simulink model "Nonlinear_compensator_regulate_position"  (R2021b)
settings: Solver=VariableStepAuto  StartTime=0.0  StopTime=10.0  RelTol=1e-3
values from neighbouring files (symbols this model uses):
  g = 9.81    [init.m]
  K = acker(A, B, P)    [Synthesis.m]
  Kr = 1/evalfr(posTf, 0)    [Synthesis.m]
  L = 2    [init.m]
  L_obs = temp'    [Synthesis.m]
  M = 5    [init.m]
  m = 1    [init.m]
  theta = pi    (= 3.14159265359)    [Synthesis.m]
  theta_perturbed = theta0 - perturbation    (= 2.99159265359)    [Linearization_comparison.m]    (also in Synthesis.m)
undefined symbols (not defined in the file or in its folder): A, B, C
settings Model: Creator=brizio  LastModifiedBy=brizio

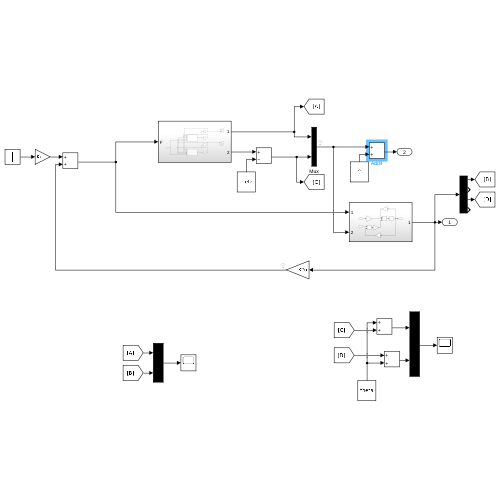
[thumbnail: Simulink's stored preview of the top-level diagram]
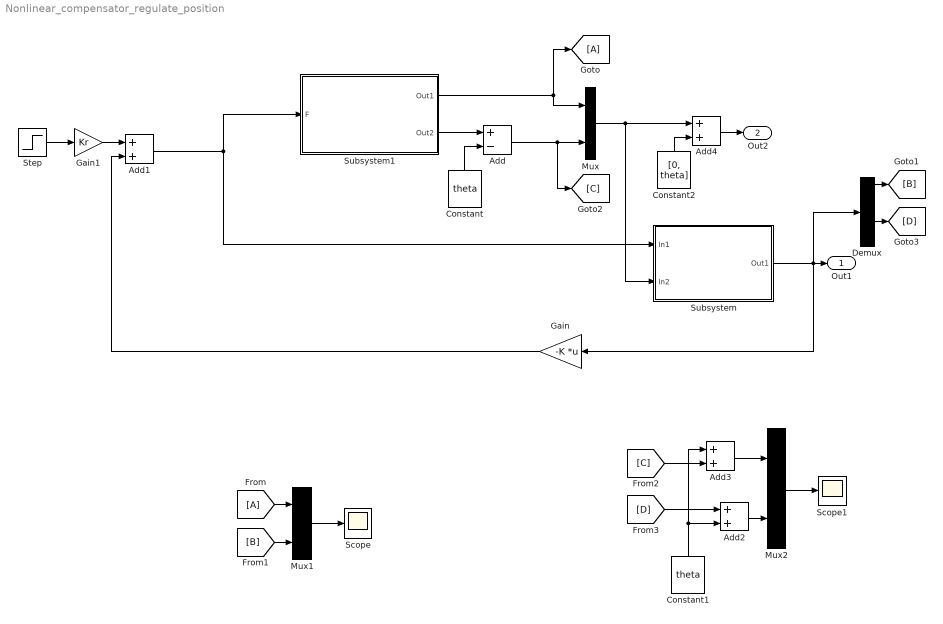
== system Nonlinear_compensator_regulate_position ==
  Add : Sum  Inputs=+-
  Add{1..4} (4 alike) : Sum
  Constant : Constant  Value=theta
  Constant1 : Constant  Value=theta
  Constant2 : Constant  Value=[0, theta]
  Demux : Demux
  Gain : Gain  Gain=-K  Multiplication=Matrix(K*u)
  Gain1 : Gain  Gain=Kr
  Mux : Mux  Inputs=2
  Mux1 : Mux  Inputs=2
  Mux2 : Mux  Inputs=2
  Scope : Scope
  Scope1 : Scope
  Step : Step  SampleTime=0
  Subsystem : Subsystem
  Subsystem1 : Subsystem
  Out1 : Outport
  Out2 : Outport  Port=2
  wires:
  Constant/1 -> Add/2
  Add2/1 -> Mux2/2
  [C] -> Add3/2
  [A] -> Mux1/1
  Add1/1 -> Subsystem1/1(F), Subsystem/1(In1)
  Add3/1 -> Mux2/1
  [B] -> Mux1/2
  Subsystem1/1(Out1) -> [A], Mux/1
  Add/1 -> [C], Mux/2
  Mux/1 -> Add4/1, Subsystem/2(In2)
  Demux/1 -> [B]
  Mux2/1 -> Scope1/1
  Subsystem/1(Out1) -> Gain/1, Out1/1, Demux/1
  [D] -> Add2/1
  Constant1/1 -> Add2/2, Add3/1
  Gain/1 -> Add1/2
  Subsystem1/2(Out2) -> Add/1
  Demux/3 -> [D]
  Mux1/1 -> Scope/1
  Gain1/1 -> Add1/1
  Step/1 -> Gain1/1
  Constant2/1 -> Add4/2
  Add4/1 -> Out2/1

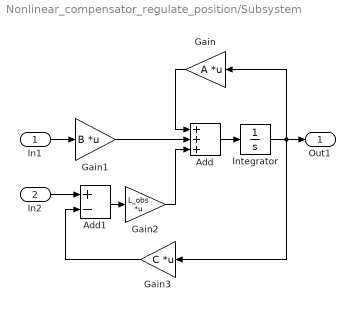
== system Nonlinear_compensator_regulate_position/Subsystem ==
  In1 : Inport
  In2 : Inport  Port=2
  Add : Sum  Inputs=+++
  Add1 : Sum  Inputs=+-
  Gain : Gain  Gain=A  Multiplication=Matrix(K*u)
  Gain1 : Gain  Gain=B  Multiplication=Matrix(K*u)
  Gain2 : Gain  Gain=L_obs  Multiplication=Matrix(K*u)
  Gain3 : Gain  Gain=C  Multiplication=Matrix(K*u)
  Integrator : Integrator
  Out1 : Outport
  wires:
  Add/1 -> Integrator/1
  In1/1 -> Gain1/1
  Gain/1 -> Add/1
  Gain1/1 -> Add/2
  Gain2/1 -> Add/3
  Add1/1 -> Gain2/1
  In2/1 -> Add1/1
  Gain3/1 -> Add1/2
  Integrator/1 -> Gain3/1, Gain/1, Out1/1

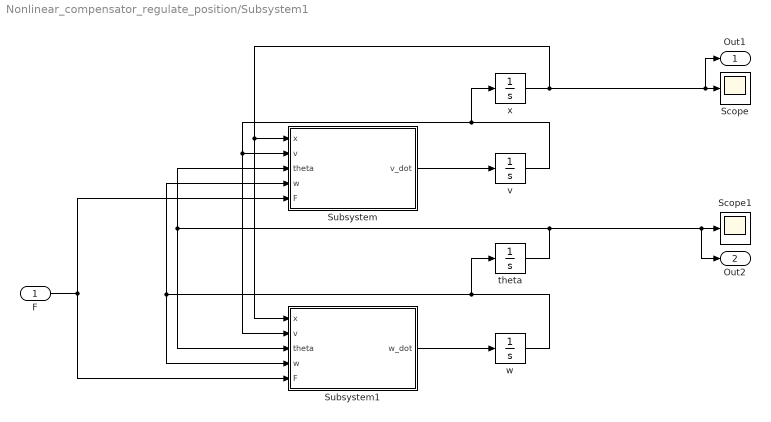
== system Nonlinear_compensator_regulate_position/Subsystem1 ==
  F : Inport
  Scope : Scope
  Scope1 : Scope
  Subsystem : Subsystem
  Subsystem1 : Subsystem
  theta : Integrator  InitialCondition=theta_perturbed
  v : Integrator
  w : Integrator
  x : Integrator
  Out1 : Outport
  Out2 : Outport  Port=2
  wires:
  theta/1 -> Out2/1, Scope1/1, Subsystem/3(theta), Subsystem1/3(theta)
  Subsystem1/1(w_dot) -> w/1
  x/1 -> Out1/1, Scope/1, Subsystem1/1(x), Subsystem/1(x)
  w/1 -> Subsystem1/4(w), Subsystem/4(w), theta/1
  F/1 -> Subsystem/5(F), Subsystem1/5(F)
  Subsystem/1(v_dot) -> v/1
  v/1 -> Subsystem/2(v), Subsystem1/2(v), x/1

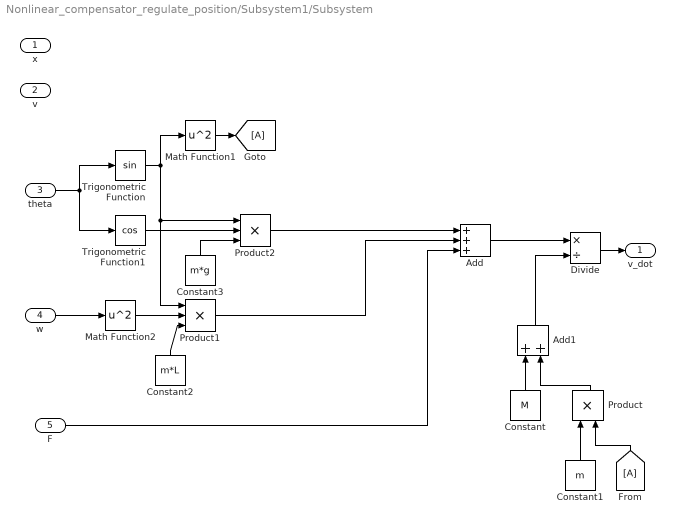
== system Nonlinear_compensator_regulate_position/Subsystem1/Subsystem ==
  x : Inport
  v : Inport  Port=2
  theta : Inport  Port=3
  w : Inport  Port=4
  F : Inport  Port=5
  Add : Sum  Inputs=+++
  Add1 : Sum
  Constant : Constant  Value=M
  Constant1 : Constant  Value=m
  Constant2 : Constant  Value=m*L
  Constant3 : Constant  Value=m*g
  Divide : Product  Inputs=*/
  Math Function1 : Math  Operator=square  SaturateOnIntegerOverflow=on
  Math Function2 : Math  Operator=square  SaturateOnIntegerOverflow=on
  Product : Product
  Product1 : Product  Inputs=3
  Product2 : Product  Inputs=3
  Trigonometric Function : Trigonometry
  Trigonometric Function1 : Trigonometry  Operator=cos
  v_dot : Outport
  wires:
  Divide/1 -> v_dot/1
  Add1/1 -> Divide/2
  Constant/1 -> Add1/1
  Product/1 -> Add1/2
  theta/1 -> Trigonometric Function1/1, Trigonometric Function/1
  Trigonometric Function/1 -> Product1/1, Product2/1, Math Function1/1
  w/1 -> Math Function2/1
  Math Function1/1 -> [A]
  [A] -> Product/2
  Constant1/1 -> Product/1
  Math Function2/1 -> Product1/2
  Constant2/1 -> Product1/3
  Add/1 -> Divide/1
  Trigonometric Function1/1 -> Product2/2
  Constant3/1 -> Product2/3
  Product1/1 -> Add/2
  Product2/1 -> Add/1
  F/1 -> Add/3

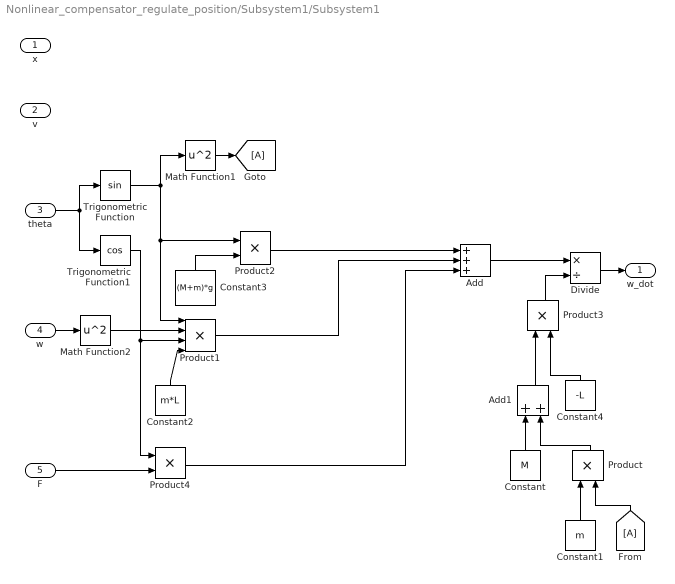
== system Nonlinear_compensator_regulate_position/Subsystem1/Subsystem1 ==
  x : Inport
  v : Inport  Port=2
  theta : Inport  Port=3
  w : Inport  Port=4
  F : Inport  Port=5
  Add : Sum  Inputs=+++
  Add1 : Sum
  Constant : Constant  Value=M
  Constant1 : Constant  Value=m
  Constant2 : Constant  Value=m*L
  Constant3 : Constant  Value=(M+m)*g
  Constant4 : Constant  Value=-L
  Divide : Product  Inputs=*/
  Math Function1 : Math  Operator=square  SaturateOnIntegerOverflow=on
  Math Function2 : Math  Operator=square  SaturateOnIntegerOverflow=on
  Product{,2..4} (4 alike) : Product
  Product1 : Product  Inputs=4
  Trigonometric Function : Trigonometry
  Trigonometric Function1 : Trigonometry  Operator=cos
  w_dot : Outport
  wires:
  Divide/1 -> w_dot/1
  Constant/1 -> Add1/1
  Product/1 -> Add1/2
  theta/1 -> Trigonometric Function1/1, Trigonometric Function/1
  Trigonometric Function/1 -> Product1/1, Product2/1, Math Function1/1
  w/1 -> Math Function2/1
  Math Function1/1 -> [A]
  [A] -> Product/2
  Constant1/1 -> Product/1
  Math Function2/1 -> Product1/2
  Add/1 -> Divide/1
  Trigonometric Function1/1 -> Product1/3, Product4/1
  Constant3/1 -> Product2/2
  Product1/1 -> Add/2
  Product2/1 -> Add/1
  Add1/1 -> Product3/1
  Product3/1 -> Divide/2
  Constant4/1 -> Product3/2
  F/1 -> Product4/2
  Product4/1 -> Add/3
  Constant2/1 -> Product1/4
